simulink model "main_model"  (R2023a)
settings: Solver=ode15s  StartTime=0.0  StopTime=4  FixedStep=0.0001  RelTol=1e-3  AbsTol=1e-3  EnableMultiTasking=on
model workspace (MAT data in the model file):
  C_Gimbal = 0.5
  C_IAP = 0.01
  K_Gimbal = 0
  K_IAP = 200
  a = 1
  b = 1
  muscle_color = [0 0 1]
  muscle_radius = 1
undefined symbols (not defined in the file): X, Y, Z
libraries: nesl_utility x346, sm_lib x329, simulink_extras x33
(part 5 of 11)

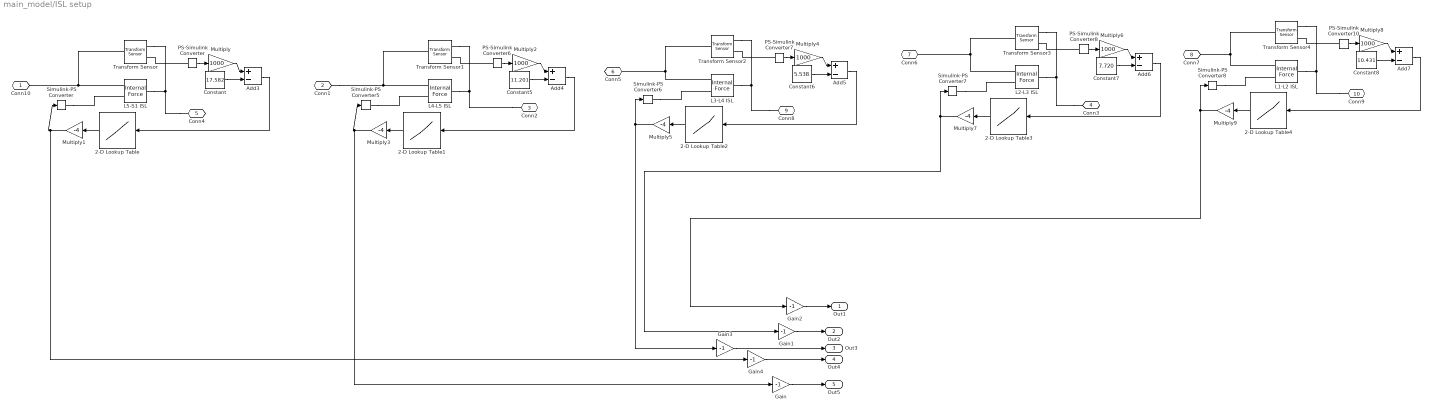
== system main_model/ISL setup ==
  2-D Lookup Table : Lookup_n-D  NumberOfTableDimensions=1  BreakpointsForDimension1=[0;0.1802;1.802;3.604;10.812]  BreakpointsForDimension2=[1:3]  Table=[0;0;4.82625;10.53;48.2625]  InternalRulePriority=Speed  RndMeth=Simplest
  2-D Lookup Table1 : Lookup_n-D  NumberOfTableDimensions=1  BreakpointsForDimension1=[0;0.1802;1.802;3.604;10.812]  BreakpointsForDimension2=[1:3]  Table=[0;0;4.82625;10.53;48.2625]  InternalRulePriority=Speed  RndMeth=Simplest
  2-D Lookup Table2 : Lookup_n-D  NumberOfTableDimensions=1  BreakpointsForDimension1=[0;0.054;0.54;1.08;3.24]  BreakpointsForDimension2=[1:3]  Table=[0;0;4.82625;10.53;48.2625]  InternalRulePriority=Speed  RndMeth=Simplest
  2-D Lookup Table3 : Lookup_n-D  NumberOfTableDimensions=1  BreakpointsForDimension1=[0;0.071;0.71;1.42;4.26]  BreakpointsForDimension2=[1:3]  Table=[0;0;4.82625;10.53;48.2625]  InternalRulePriority=Speed  RndMeth=Simplest
  2-D Lookup Table4 : Lookup_n-D  NumberOfTableDimensions=1  BreakpointsForDimension1=[0;0.105;1.05;2.1;6.3]  BreakpointsForDimension2=[1:3]  Table=[0;0;4.82625;10.53;48.2625]  InternalRulePriority=Speed  RndMeth=Simplest
  Add{3..7} (5 alike) : Sum  Inputs=+-
  Constant : Constant  Value=17.582
  Constant5 : Constant  Value=11.201
  Constant6 : Constant  Value=5.538
  Constant7 : Constant  Value=7.720
  Constant8 : Constant  Value=10.431
  Gain{,1..4} (5 alike) : Gain  Gain=-1
  L1-L2 ISL : sm_lib/Forces and Torques/Internal Force
  L2-L3 ISL : sm_lib/Forces and Torques/Internal Force
  L3-L4 ISL : sm_lib/Forces and Torques/Internal Force
  L4-L5 ISL : sm_lib/Forces and Torques/Internal Force
  L5-S1 ISL : sm_lib/Forces and Torques/Internal Force
  Multiply{,2,4,6,8} (5 alike) : Gain  Gain=1000
  Multiply{1,3,5,7,9} (5 alike) : Gain  Gain=-4
  PS-Simulink Converter{,6..8,10} (5 alike) : nesl_utility/PS-Simulink Converter  PhysicalDomain=network_engine_domain  SubClassName=ps_output  LeftPortType=input  RightPortType=output  PseudoPeriodic=off  Frequencies=[]  VectorFormat=inherit  Unit=inherit  AffineConversion=off
  Simulink-PS Converter{,5..8} (5 alike) : nesl_utility/Simulink-PS Converter  PhysicalDomain=network_engine_domain  SubClassName=ps_input  LeftPortType=input  RightPortType=output  PseudoPeriodic=off  Frequencies=[]  NoiseDistribution=none  NoiseParameters=[]  Unit=1  AffineConversion=off  FilteringAndDerivatives=provide  SimscapeFilterOrder=1  InputFilterTimeConstant=0.001  UdotUserProvided=0
  Transform Sensor{,1..4} (5 alike) : sm_lib/Frames and Transforms/Transform Sensor  MeasurementFrame=World  RotationSequence=XYX  SenseAngle=off  SenseAxis=off  SenseQ=off  SenseR=off  SenseRotationSequence=off  SenseOmegaX=off  SenseOmegaY=off  SenseOmegaZ=off  SenseQDot=off  SenseRDot=off  SenseRotationSequenceDot=off  SenseAlphaX=off  SenseAlphaY=off  SenseAlphaZ=off  SenseQDDot=off  SenseRDDot=off  SenseX=off  SenseY=off  SenseZ=off  SenseRad=off  SenseAzim=off  SenseDist=on  SenseInc=off  SenseXDot=off  SenseYDot=off  SenseZDot=off  SenseRadDot=off  SenseAzimDot=off  SenseDistDot=off  SenseIncDot=off  SenseXDDot=off  SenseYDDot=off  SenseZDDot=off  SenseRadDDot=off  SenseAzimDDot=off  SenseDistDDot=off  SenseIncDDot=off
  Conn10 : PMIOPort  Side=Left
  Conn1 : PMIOPort  Port=2  Side=Left
  Conn2 : PMIOPort  Port=3  Side=Left
  Conn3 : PMIOPort  Port=4  Side=Left
  Conn4 : PMIOPort  Port=5  Side=Left
  Conn5 : PMIOPort  Port=6  Side=Left
  Conn6 : PMIOPort  Port=7  Side=Left
  Conn7 : PMIOPort  Port=8  Side=Left
  Conn8 : PMIOPort  Port=9  Side=Left
  Conn9 : PMIOPort  Port=10  Side=Left
  Out1 : Outport
  Out2 : Outport  Port=2
  Out3 : Outport  Port=3
  Out4 : Outport  Port=4
  Out5 : Outport  Port=5
  wires:
  Gain/1 -> Out5/1
  Gain4/1 -> Out4/1
  Gain3/1 -> Out3/1
  Gain1/1 -> Out2/1
  Gain2/1 -> Out1/1
  Multiply5/1 -> Simulink-PS Converter6/1, Gain3/1
  2-D Lookup Table4/1 -> Multiply9/1
  PS-Simulink Converter/1 -> Multiply/1
  2-D Lookup Table3/1 -> Multiply7/1
  Add6/1 -> 2-D Lookup Table3/1
  Multiply/1 -> Add3/1
  2-D Lookup Table/1 -> Multiply1/1
  Constant7/1 -> Add6/2
  Multiply1/1 -> Simulink-PS Converter/1, Gain4/1
  Multiply8/1 -> Add7/1
  PS-Simulink Converter6/1 -> Multiply2/1
  2-D Lookup Table2/1 -> Multiply5/1
  Constant/1 -> Add3/2
  2-D Lookup Table1/1 -> Multiply3/1
  Constant6/1 -> Add5/2
  Multiply3/1 -> Simulink-PS Converter5/1, Gain/1
  Add4/1 -> 2-D Lookup Table1/1
  Multiply9/1 -> Simulink-PS Converter8/1, Gain2/1
  Constant5/1 -> Add4/2
  Multiply7/1 -> Simulink-PS Converter7/1, Gain1/1
  Multiply4/1 -> Add5/1
  Add3/1 -> 2-D Lookup Table/1
  Multiply2/1 -> Add4/1
  Add7/1 -> 2-D Lookup Table4/1
  PS-Simulink Converter7/1 -> Multiply4/1
  Constant8/1 -> Add7/2
  Add5/1 -> 2-D Lookup Table2/1
  PS-Simulink Converter10/1 -> Multiply8/1
  Multiply6/1 -> Add6/1
  PS-Simulink Converter8/1 -> Multiply6/1
  connections:
  Simulink-PS Converter5/RConn1 -- L4-L5 ISL/LConn2
  PS-Simulink Converter10/LConn1 -- Transform Sensor4/RConn2
  PS-Simulink Converter6/LConn1 -- Transform Sensor1/RConn2
  Simulink-PS Converter/RConn1 -- L5-S1 ISL/LConn2
  PS-Simulink Converter7/LConn1 -- Transform Sensor2/RConn2
  PS-Simulink Converter/LConn1 -- Transform Sensor/RConn2
  Simulink-PS Converter6/RConn1 -- L3-L4 ISL/LConn2
  PS-Simulink Converter8/LConn1 -- Transform Sensor3/RConn2
  Simulink-PS Converter8/RConn1 -- L1-L2 ISL/LConn2
  Conn5/RConn1 -- Transform Sensor2/LConn1 -- L3-L4 ISL/LConn1
  Conn4/RConn1 -- Transform Sensor/RConn1 -- L5-S1 ISL/RConn1
  Conn6/RConn1 -- Transform Sensor3/LConn1 -- L2-L3 ISL/LConn1
  Conn9/RConn1 -- Transform Sensor4/RConn1 -- L1-L2 ISL/RConn1
  Simulink-PS Converter7/RConn1 -- L2-L3 ISL/LConn2
  Conn3/RConn1 -- Transform Sensor3/RConn1 -- L2-L3 ISL/RConn1
  Conn7/RConn1 -- Transform Sensor4/LConn1 -- L1-L2 ISL/LConn1
  Conn8/RConn1 -- Transform Sensor2/RConn1 -- L3-L4 ISL/RConn1
  Conn1/RConn1 -- Transform Sensor1/LConn1 -- L4-L5 ISL/LConn1
  Conn2/RConn1 -- Transform Sensor1/RConn1 -- L4-L5 ISL/RConn1
  Conn10/RConn1 -- Transform Sensor/LConn1 -- L5-S1 ISL/LConn1

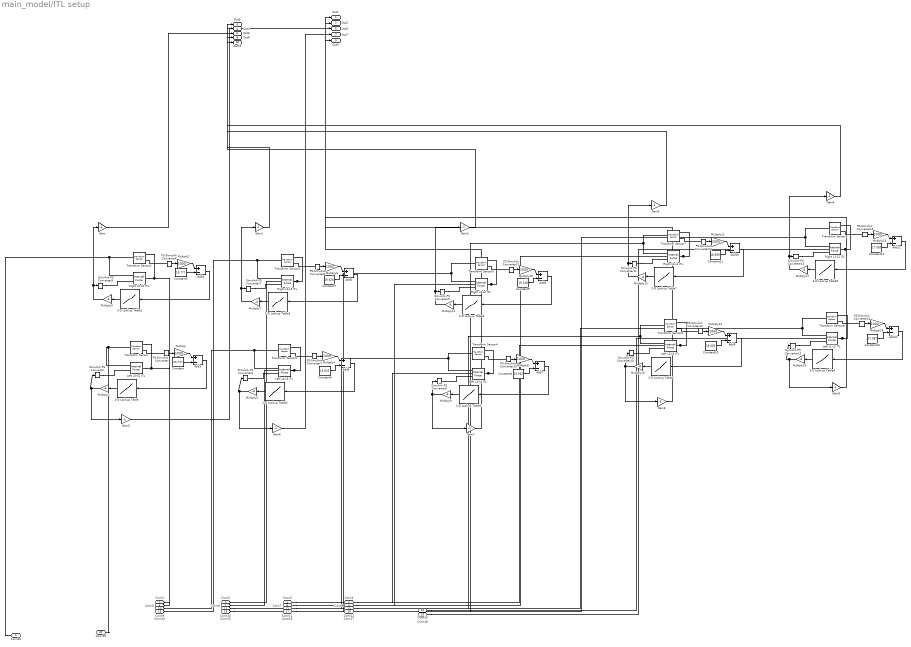
== system main_model/ITL setup ==
  2-D Lookup Table : Lookup_n-D  NumberOfTableDimensions=1  BreakpointsForDimension1=[0;0.178;2.67;3.916;5.34]  BreakpointsForDimension2=[1:3]  Table=[0;0;3;7.5;30]  InternalRulePriority=Speed  RndMeth=Simplest
  2-D Lookup Table1 : Lookup_n-D  NumberOfTableDimensions=1  BreakpointsForDimension1=[0;0.178;2.67;3.916;5.34]  BreakpointsForDimension2=[1:3]  Table=[0;0;3;7.5;30]  InternalRulePriority=Speed  RndMeth=Simplest
  2-D Lookup Table2 : Lookup_n-D  NumberOfTableDimensions=1  BreakpointsForDimension1=[0;0.213;3.195;4.686;6.39]  BreakpointsForDimension2=[1:3]  Table=[0;0;3;7.5;30]  InternalRulePriority=Speed  RndMeth=Simplest
  2-D Lookup Table3 : Lookup_n-D  NumberOfTableDimensions=1  BreakpointsForDimension1=[0;0.213;3.195;4.686;6.39]  BreakpointsForDimension2=[1:3]  Table=[0;0;3;7.5;30]  InternalRulePriority=Speed  RndMeth=Simplest
  2-D Lookup Table4 : Lookup_n-D  NumberOfTableDimensions=1  BreakpointsForDimension1=[0;0.1985;2.9775;4.367;5.955]  BreakpointsForDimension2=[1:3]  Table=[0;0;3;7.5;30]  InternalRulePriority=Speed  RndMeth=Simplest
  2-D Lookup Table5 : Lookup_n-D  NumberOfTableDimensions=1  BreakpointsForDimension1=[0;0.1985;2.9775;4.367;5.955]  BreakpointsForDimension2=[1:3]  Table=[0;0;3;7.5;30]  InternalRulePriority=Speed  RndMeth=Simplest
  2-D Lookup Table6 : Lookup_n-D  NumberOfTableDimensions=1  BreakpointsForDimension1=[0;0.2084;3.126;4.5848;6.252]  BreakpointsForDimension2=[1:3]  Table=[0;0;3;7.5;30]  InternalRulePriority=Speed  RndMeth=Simplest
  2-D Lookup Table7 : Lookup_n-D  NumberOfTableDimensions=1  BreakpointsForDimension1=[0;0.2084;3.126;4.5848;6.252]  BreakpointsForDimension2=[1:3]  Table=[0;0;3;7.5;30]  InternalRulePriority=Speed  RndMeth=Simplest
  2-D Lookup Table8 : Lookup_n-D  NumberOfTableDimensions=1  BreakpointsForDimension1=[0;0.1966;2.949;4.3252;5.898]  BreakpointsForDimension2=[1:3]  Table=[0;0;3;7.5;30]  InternalRulePriority=Speed  RndMeth=Simplest
  2-D Lookup Table9 : Lookup_n-D  NumberOfTableDimensions=1  BreakpointsForDimension1=[0;0.1966;2.949;4.3252;5.898]  BreakpointsForDimension2=[1:3]  Table=[0;0;3;7.5;30]  InternalRulePriority=Speed  RndMeth=Simplest
  Add{3..12} (10 alike) : Sum  Inputs=+-
  Constant : Constant  Value=15.777
  Constant10 : Constant  Value=18.659
  Constant11 : Constant  Value=18.659
  Constant12 : Constant  Value=17.087
  Constant13 : Constant  Value=17.087
  Constant5 : Constant  Value=15.777
  Constant6 : Constant  Value=19.625
  Constant7 : Constant  Value=19.625
  Constant8 : Constant  Value=19.562
  Constant9 : Constant  Value=19.248
  Gain{,1..9} (10 alike) : Gain  Gain=-1
  Left L1-L2 ITL : sm_lib/Forces and Torques/Internal Force
  Left L2-L3 ITL : sm_lib/Forces and Torques/Internal Force
  Left L3-L4 ITL : sm_lib/Forces and Torques/Internal Force
  Left L4-L5 ITL : sm_lib/Forces and Torques/Internal Force
  Left L5-S1 ITL : sm_lib/Forces and Torques/Internal Force
  Multiply{,2,4,6,8,10,12,14,16,18} (10 alike) : Gain  Gain=1000
  Multiply{1,3,5,7,9,11,13,15,17,19} (10 alike) : Gain  Gain=-4
  PS-Simulink Converter{,6..8,10..15} (10 alike) : nesl_utility/PS-Simulink Converter  PhysicalDomain=network_engine_domain  SubClassName=ps_output  LeftPortType=input  RightPortType=output  PseudoPeriodic=off  Frequencies=[]  VectorFormat=inherit  Unit=inherit  AffineConversion=off
  Right L1-L2 ITL : sm_lib/Forces and Torques/Internal Force
  Right L2-L3 ITL : sm_lib/Forces and Torques/Internal Force
  Right L3-L4 ITL : sm_lib/Forces and Torques/Internal Force
  Right L4-L5 ITL : sm_lib/Forces and Torques/Internal Force
  Right L5-S1 ITL : sm_lib/Forces and Torques/Internal Force
  Simulink-PS Converter{,5..13} (10 alike) : nesl_utility/Simulink-PS Converter  PhysicalDomain=network_engine_domain  SubClassName=ps_input  LeftPortType=input  RightPortType=output  PseudoPeriodic=off  Frequencies=[]  NoiseDistribution=none  NoiseParameters=[]  Unit=1  AffineConversion=off  FilteringAndDerivatives=provide  SimscapeFilterOrder=1  InputFilterTimeConstant=0.001  UdotUserProvided=0
  Transform Sensor{,1..9} (10 alike) : sm_lib/Frames and Transforms/Transform Sensor  MeasurementFrame=World  RotationSequence=XYX  SenseAngle=off  SenseAxis=off  SenseQ=off  SenseR=off  SenseRotationSequence=off  SenseOmegaX=off  SenseOmegaY=off  SenseOmegaZ=off  SenseQDot=off  SenseRDot=off  SenseRotationSequenceDot=off  SenseAlphaX=off  SenseAlphaY=off  SenseAlphaZ=off  SenseQDDot=off  SenseRDDot=off  SenseX=off  SenseY=off  SenseZ=off  SenseRad=off  SenseAzim=off  SenseDist=on  SenseInc=off  SenseXDot=off  SenseYDot=off  SenseZDot=off  SenseRadDot=off  SenseAzimDot=off  SenseDistDot=off  SenseIncDot=off  SenseXDDot=off  SenseYDDot=off  SenseZDDot=off  SenseRadDDot=off  SenseAzimDDot=off  SenseDistDDot=off  SenseIncDDot=off
  Conn20 : PMIOPort  Side=Left
  Conn1 : PMIOPort  Port=2  Side=Left
  Conn2 : PMIOPort  Port=3  Side=Left
  Conn3 : PMIOPort  Port=4  Side=Left
  Conn4 : PMIOPort  Port=5  Side=Left
  Conn5 : PMIOPort  Port=6  Side=Left
  Conn6 : PMIOPort  Port=7  Side=Left
  Conn7 : PMIOPort  Port=8  Side=Left
  Conn8 : PMIOPort  Port=9  Side=Left
  Conn9 : PMIOPort  Port=10  Side=Left
  Conn10 : PMIOPort  Port=11  Side=Left
  Conn11 : PMIOPort  Port=12  Side=Left
  Conn12 : PMIOPort  Port=13  Side=Left
  Conn13 : PMIOPort  Port=14  Side=Left
  Conn14 : PMIOPort  Port=15  Side=Left
  Conn15 : PMIOPort  Port=16  Side=Left
  Conn16 : PMIOPort  Port=17  Side=Left
  Conn17 : PMIOPort  Port=18  Side=Left
  Conn18 : PMIOPort  Port=19  Side=Left
  Conn19 : PMIOPort  Port=20  Side=Left
  Out1 : Outport
  Out2 : Outport  Port=2
  Out3 : Outport  Port=3
  Out4 : Outport  Port=4
  Out5 : Outport  Port=5
  Out6 : Outport  Port=6
  Out7 : Outport  Port=7
  Out8 : Outport  Port=8
  Out9 : Outport  Port=9
  Out10 : Outport  Port=10
  wires:
  Gain5/1 -> Out5/1
  Gain6/1 -> Out7/1
  Gain8/1 -> Out2/1
  Gain9/1 -> Out1/1
  Gain/1 -> Out6/1
  Add12/1 -> 2-D Lookup Table8/1
  Gain3/1 -> Out4/1
  PS-Simulink Converter10/1 -> Multiply8/1
  Gain7/1 -> Out9/1
  2-D Lookup Table9/1 -> Multiply17/1
  PS-Simulink Converter7/1 -> Multiply4/1
  Constant8/1 -> Add7/2
  Gain4/1 -> Out3/1
  Constant11/1 -> Add10/2
  2-D Lookup Table3/1 -> Multiply7/1
  Multiply7/1 -> Simulink-PS Converter7/1, Gain1/1
  2-D Lookup Table8/1 -> Multiply19/1
  Multiply6/1 -> Add6/1
  Add8/1 -> 2-D Lookup Table5/1
  2-D Lookup Table/1 -> Multiply1/1
  Multiply4/1 -> Add5/1
  Add6/1 -> 2-D Lookup Table3/1
  Gain1/1 -> Out8/1
  Multiply16/1 -> Add11/1
  Multiply15/1 -> Simulink-PS Converter10/1, Gain8/1
  PS-Simulink Converter6/1 -> Multiply2/1
  Constant12/1 -> Add12/2
  Add3/1 -> 2-D Lookup Table/1
  Constant7/1 -> Add6/2
  2-D Lookup Table1/1 -> Multiply3/1
  2-D Lookup Table2/1 -> Multiply5/1
  Multiply8/1 -> Add7/1
  Constant9/1 -> Add8/2
  Add4/1 -> 2-D Lookup Table1/1
  Constant6/1 -> Add5/2
  Add11/1 -> 2-D Lookup Table9/1
  PS-Simulink Converter15/1 -> Multiply16/1
  PS-Simulink Converter13/1 -> Multiply12/1
  2-D Lookup Table4/1 -> Multiply9/1
  Constant5/1 -> Add4/2
  2-D Lookup Table7/1 -> Multiply13/1
  Multiply14/1 -> Add9/1
  Multiply/1 -> Add3/1
  PS-Simulink Converter8/1 -> Multiply6/1
  Add10/1 -> 2-D Lookup Table7/1
  Constant/1 -> Add3/2
  Gain2/1 -> Out10/1
  Multiply13/1 -> Simulink-PS Converter11/1, Gain3/1
  Multiply12/1 -> Add10/1
  PS-Simulink Converter14/1 -> Multiply18/1
  Multiply10/1 -> Add8/1
  Multiply17/1 -> Simulink-PS Converter13/1, Gain4/1
  PS-Simulink Converter/1 -> Multiply/1
  2-D Lookup Table5/1 -> Multiply11/1
  Multiply2/1 -> Add4/1
  Multiply11/1 -> Simulink-PS Converter9/1, Gain2/1
  Multiply19/1 -> Simulink-PS Converter12/1, Gain9/1
  Add9/1 -> 2-D Lookup Table6/1
  Multiply18/1 -> Add12/1
  Constant10/1 -> Add9/2
  PS-Simulink Converter11/1 -> Multiply10/1
  Multiply1/1 -> Simulink-PS Converter/1, Gain5/1
  Multiply3/1 -> Simulink-PS Converter5/1, Gain/1
  Multiply9/1 -> Gain7/1, Simulink-PS Converter8/1
  Add5/1 -> 2-D Lookup Table2/1
  Add7/1 -> 2-D Lookup Table4/1
  Constant13/1 -> Add11/2
  PS-Simulink Converter12/1 -> Multiply14/1
  Multiply5/1 -> Simulink-PS Converter6/1, Gain6/1
  2-D Lookup Table6/1 -> Multiply15/1
  connections:
  PS-Simulink Converter8/LConn1 -- Transform Sensor3/RConn2
  PS-Simulink Converter11/LConn1 -- Transform Sensor5/RConn2
  Simulink-PS Converter12/RConn1 -- Left L1-L2 ITL/LConn2
  Conn14/RConn1 -- Right L4-L5 ITL/LConn1 -- Transform Sensor3/LConn1
  Simulink-PS Converter7/RConn1 -- Right L4-L5 ITL/LConn2
  Conn1/RConn1 -- Transform Sensor/RConn1 -- Left L5-S1 ITL/RConn1
  Conn10/RConn1 -- Left L3-L4 ITL/LConn1 -- Transform Sensor4/LConn1
  Simulink-PS Converter11/RConn1 -- Right L2-L3 ITL/LConn2
  Simulink-PS Converter10/RConn1 -- Left L2-L3 ITL/LConn2
  Conn12/RConn1 -- Left L1-L2 ITL/LConn1 -- Transform Sensor8/LConn1
  Simulink-PS Converter9/RConn1 -- Right L3-L4 ITL/LConn2
  PS-Simulink Converter7/LConn1 -- Transform Sensor2/RConn2
  PS-Simulink Converter6/LConn1 -- Transform Sensor1/RConn2
  Conn8/RConn1 -- Transform Sensor7/RConn1 -- Right L2-L3 ITL/RConn1
  PS-Simulink Converter14/LConn1 -- Transform Sensor8/RConn2
  Simulink-PS Converter13/RConn1 -- Right L1-L2 ITL/LConn2
  Conn3/RConn1 -- Transform Sensor4/RConn1 -- Left L3-L4 ITL/RConn1
  Conn18/RConn1 -- Transform Sensor9/RConn1 -- Right L1-L2 ITL/RConn1
  PS-Simulink Converter15/LConn1 -- Transform Sensor9/RConn2
  Simulink-PS Converter6/RConn1 -- Left L4-L5 ITL/LConn2
  Conn17/RConn1 -- Right L1-L2 ITL/LConn1 -- Transform Sensor9/LConn1
  Conn15/RConn1 -- Right L3-L4 ITL/LConn1 -- Transform Sensor5/LConn1
  PS-Simulink Converter12/LConn1 -- Transform Sensor6/RConn2
  Conn7/RConn1 -- Transform Sensor5/RConn1 -- Right L3-L4 ITL/RConn1
  Simulink-PS Converter5/RConn1 -- Right L5-S1 ITL/LConn2
  Conn13/RConn1 -- Transform Sensor8/RConn1 -- Left L1-L2 ITL/RConn1
  PS-Simulink Converter/LConn1 -- Transform Sensor/RConn2
  Conn11/RConn1 -- Left L2-L3 ITL/LConn1 -- Transform Sensor6/LConn1
  Simulink-PS Converter8/RConn1 -- Left L3-L4 ITL/LConn2
  Conn5/RConn1 -- Transform Sensor1/RConn1 -- Right L5-S1 ITL/RConn1
  Conn19/RConn1 -- Transform Sensor/LConn1 -- Left L5-S1 ITL/LConn1
  Conn4/RConn1 -- Transform Sensor6/RConn1 -- Left L2-L3 ITL/RConn1
  Conn20/RConn1 -- Right L5-S1 ITL/LConn1 -- Transform Sensor1/LConn1
  Conn9/RConn1 -- Left L4-L5 ITL/LConn1 -- Transform Sensor2/LConn1
  Conn16/RConn1 -- Right L2-L3 ITL/LConn1 -- Transform Sensor7/LConn1
  Conn6/RConn1 -- Transform Sensor2/RConn1 -- Left L4-L5 ITL/RConn1
  Conn2/RConn1 -- Transform Sensor3/RConn1 -- Right L4-L5 ITL/RConn1
  Simulink-PS Converter/RConn1 -- Left L5-S1 ITL/LConn2
  PS-Simulink Converter13/LConn1 -- Transform Sensor7/RConn2
  PS-Simulink Converter10/LConn1 -- Transform Sensor4/RConn2

== system main_model/L1 ==
  AR torque feedback L4 : Subsystem
  FE torque feedback L4 : Subsystem
  File Solid : sm_lib/Body Elements/File Solid  ExtGeomFileName=C:\Users\siril\OneDrive\Desktop\TIM-Control\Matlab\Simscape models\CAD - with COM\SymmetricModel\draft7\L1.step  UnitType=FromFile  ExtGeomFileUnits=m  StepReaderType=HEX  ExportConvexHullGeometry=off  InertiaType=CalculateFromGeometry  Mass=1  MassUnits=kg  CenterOfMass=[0 0 0]  CenterOfMassUnits=m  MomentsOfInertia=[1 1 1]  MomentsOfInertiaUnits=kg*m^2  ProductsOfInertia=[0 0 0]  ProductsOfInertiaUnits=kg*m^2  BasedOnType=Density  Density=0.182  DensityUnits=g/cm^3  DoExposeReferenceFrame=on  SerializedFrames=<Frames><Frame><Id>Frame1</Id><Value><Name>To L2</Name><Origin><Source>GeometricFeature</Source><FeatureName>planar surface 2992</FeatureName></Origin><PrimaryAxis><DefinedDirection>+Z</DefinedDirection><Source>GeometricFeature</Source><SourceDirection>+Z</SourceDirection><FeatureName>planar surface 2992</FeatureName></PrimaryAxis><SecondaryAxis><DefinedDirection>+X</DefinedDirection><Source>ReferenceFrame</Source><SourceDirection>+X</SourceDirection><FeatureName></FeatureName></SecondaryAxis></Value></Frame><Frame><Id>Frame2</Id><Value><Name>To T12</Name><Origin><Source>GeometricFeature</Source><FeatureName>segment 4586</FeatureName></Origin><PrimaryAxis><DefinedDirection>+Z</DefinedDirection><Source>GeometricFeature</Source><SourceDirection>+Z</SourceDirection><FeatureName>planar surface 2965</FeatureName></PrimaryAxis><SecondaryAxis><DefinedDirection>+X</DefinedDirection><Source>ReferenceFrame</Source><SourceDirection>+X</SourceDirection><FeatureName></FeatureName></SecondaryAxis></Value></Frame><Frame><Id>Frame3</Id><Value><Name>L1 COM</Name><Origin><Source>CenterOfMassFrame</Source><FeatureName></FeatureName></Origin><PrimaryAxis><DefinedDirection>+Z</DefinedDirection><Source>ReferenceFrame</Source><SourceDirection>+Z</SourceDirection><FeatureName></FeatureName></PrimaryAxis><SecondaryAxis><DefinedDirection>+X</DefinedDirection><Source>ReferenceFrame</Source><SourceDirection>+X</SourceDirection><FeatureName></FeatureName></SecondaryAxis></Value></Frame><Frame><Id>Frame4</Id><Value><Name>L1 Abd Force</Name><Origin><Source>GeometricFeature</Source><FeatureName>point 2</FeatureName></Origin><PrimaryAxis><DefinedDirection>+Z</DefinedDirection><Source>GeometricFeature</Source><SourceDirection>+Z</SourceDirection><FeatureName>conical surface 2</FeatureName></PrimaryAxis><SecondaryAxis><DefinedDirection>+X</DefinedDirection><Source>ReferenceFrame</Source><SourceDirection>+X</SourceDirection><FeatureName></FeatureName></SecondaryAxis></Value></Frame><Frame><Id>Frame5</Id><Value><Name>To L2 ISL</Name><Origin><Source>GeometricFeature</Source><FeatureName>point 8203</FeatureName></Origin><PrimaryAxis><DefinedDirection>+Z</DefinedDirection><Source>ReferenceFrame</Source><SourceDirection>+Z</SourceDirection><FeatureName></FeatureName></PrimaryAxis><SecondaryAxis><DefinedDirection>+X</DefinedDirection><Source>ReferenceFrame</Source><SourceDirection>+X</SourceDirection><FeatureName></FeatureName></SecondaryAxis></Value></Frame><Frame><Id>Frame6</Id><Value><Name>To L2 SSL</Name><Origin><Source>GeometricFeature</Source><FeatureName>point 7953</FeatureName></Origin><PrimaryAxis><DefinedDirection>+Z</DefinedDirection><Source>ReferenceFrame</Source><SourceDirection>+Z</SourceDirection><FeatureName></FeatureName></PrimaryAxis><SecondaryAxis><DefinedDirection>+X</DefinedDirection><Source>ReferenceFrame</Source><SourceDirection>+X</SourceDirection><FeatureName></FeatureName></SecondaryAxis></Value></Frame><Frame><Id>Frame7</Id><Value><Name>To Left L2 ITL</Name><Origin><Source>GeometricFeature</Source><FeatureName>point 8094</FeatureName></Origin><PrimaryAxis><DefinedDirection>+Z</DefinedDirection><Source>ReferenceFrame</Source><SourceDirection>+Z</SourceDirection><FeatureName></FeatureName></PrimaryAxis><SecondaryAxis><DefinedDirection>+X</DefinedDirection><Source>ReferenceFrame</Source><SourceDirection>+X</SourceDirection><FeatureName></FeatureName></SecondaryAxis></Value></Frame><Frame><Id>Frame8</Id><Value><Name>To Right L2 ITL</Name><Origin><Source>GeometricFeature</Source><FeatureName>point 3432</FeatureName></Origin><PrimaryAxis><DefinedDirection>+Z</DefinedDirection><Source>ReferenceFrame</Source><SourceDirection>+Z</SourceDirection><FeatureName></FeatureName></PrimaryAxis><SecondaryAxis><DefinedDirection>+X</DefinedDirection><Source>ReferenceFrame</Source><SourceDirection>+X</SourceDirection><FeatureName></FeatureName></SecondaryAxis></Value></Frame></Frames>  GraphicType=FromGeometry  MarkerShape=Sphere  MarkerSize=10  GraphicVisPropType=SimpleVisualProperties  GraphicDiffuseColor=[0.8901961 0.85490197 0.7882353]  GraphicSpecularColor=[0.5 0.5 0.5 1.0]  GraphicAmbientColor=[0.15 0.15 0.15 1.0]  GraphicEmissiveColor=[0.0 0.0 0.0 1.0]  GraphicShininess=75  GraphicOpacity=1.0
  Gimbal Joint1 : sm_lib/Joints/Gimbal Joint  JointMode=Normal  SenseConstraintForce=off  SenseConstraintForceX=off  SenseConstraintForceY=off  SenseConstraintForceZ=off  SenseConstraintTorque=off  SenseConstraintTorqueX=off  SenseConstraintTorqueY=off  SenseConstraintTorqueZ=off  SenseTotalForce=off  SenseTotalForceX=off  SenseTotalForceY=off  SenseTotalForceZ=off  SenseTotalTorque=off  SenseTotalTorqueX=off  SenseTotalTorqueY=off  SenseTotalTorqueZ=off  CompositeWrenchDir=FollowerOnBase  CompositeWrenchFrame=BaseFrame  RxEquilibriumPosition=0  RxEquilibriumPositionUnits=deg  RxSpringStiffness=K_Gimbal  RxSpringStiffnessUnits=N*m/deg  RxDampingCoefficient=C_Gimbal  RxDampingCoefficientUnits=N*m/(deg/s)  RxTorqueActuationMode=InputTorque  RxMotionActuationMode=ComputedMotion  RxSensePosition=on  RxSenseVelocity=off  RxSenseAcceleration=off  RxSenseTorqueForce=on  RxSenseLowerLimitTorqueForce=off  RxSenseUpperLimitTorqueForce=off  RxLowerLimitSpecify=on  RxLowerLimitBound=-30  RxLowerLimitBoundUnits=deg  RxLowerLimitStiffness=10000  RxLowerLimitStiffnessUnits=N*m/deg  RxLowerLimitDamping=100  RxLowerLimitDampingUnits=N*m/(deg/s)  RxLowerLimitTransitionRegionWidth=0.1  RxLowerLimitTransitionRegionWidthUnits=deg  RxUpperLimitSpecify=on  RxUpperLimitBound=30  RxUpperLimitBoundUnits=deg  RxUpperLimitStiffness=10000  RxUpperLimitStiffnessUnits=N*m/deg  RxUpperLimitDamping=100  RxUpperLimitDampingUnits=N*m/(deg/s)  RxUpperLimitTransitionRegionWidth=0.1  RxUpperLimitTransitionRegionWidthUnits=deg  RxPositionTargetSpecify=off  RxPositionTargetPriority=High  RxPositionTargetValue=0  RxPositionTargetValueUnits=deg  RxVelocityTargetSpecify=off  RxVelocityTargetPriority=High  RxVelocityTargetValue=0  RxVelocityTargetValueUnits=deg/s  RyEquilibriumPosition=0  RyEquilibriumPositionUnits=deg  RySpringStiffness=K_Gimbal  RySpringStiffnessUnits=N*m/deg  RyDampingCoefficient=C_Gimbal  RyDampingCoefficientUnits=N*m/(deg/s)  RyTorqueActuationMode=InputTorque  RyMotionActuationMode=ComputedMotion  RySensePosition=on  RySenseVelocity=off  RySenseAcceleration=off  RySenseTorqueForce=on  RySenseLowerLimitTorqueForce=off  RySenseUpperLimitTorqueForce=off  RyLowerLimitSpecify=on  RyLowerLimitBound=-30  RyLowerLimitBoundUnits=deg  RyLowerLimitStiffness=10000  RyLowerLimitStiffnessUnits=N*m/deg  RyLowerLimitDamping=100  RyLowerLimitDampingUnits=N*m/(deg/s)  RyLowerLimitTransitionRegionWidth=0.1  RyLowerLimitTransitionRegionWidthUnits=deg  RyUpperLimitSpecify=on  RyUpperLimitBound=30  RyUpperLimitBoundUnits=deg  RyUpperLimitStiffness=10000  RyUpperLimitStiffnessUnits=N*m/deg  RyUpperLimitDamping=100  RyUpperLimitDampingUnits=N*m/(deg/s)  RyUpperLimitTransitionRegionWidth=0.1  RyUpperLimitTransitionRegionWidthUnits=deg  RyPositionTargetSpecify=off  RyPositionTargetPriority=High  RyPositionTargetValue=0  RyPositionTargetValueUnits=deg  RyVelocityTargetSpecify=off  RyVelocityTargetPriority=High  RyVelocityTargetValue=0  RyVelocityTargetValueUnits=deg/s  RzEquilibriumPosition=0  RzEquilibriumPositionUnits=deg  RzSpringStiffness=K_Gimbal  RzSpringStiffnessUnits=N*m/deg  RzDampingCoefficient=C_Gimbal  RzDampingCoefficientUnits=N*m/(deg/s)  RzTorqueActuationMode=InputTorque  RzMotionActuationMode=ComputedMotion  RzSensePosition=on  RzSenseVelocity=off  RzSenseAcceleration=off  RzSenseTorqueForce=on  RzSenseLowerLimitTorqueForce=off  RzSenseUpperLimitTorqueForce=off  RzLowerLimitSpecify=on  RzLowerLimitBound=-30  RzLowerLimitBoundUnits=deg  RzLowerLimitStiffness=10000  RzLowerLimitStiffnessUnits=N*m/deg  RzLowerLimitDamping=100  RzLowerLimitDampingUnits=N*m/(deg/s)  RzLowerLimitTransitionRegionWidth=0.1  RzLowerLimitTransitionRegionWidthUnits=deg  RzUpperLimitSpecify=on  RzUpperLimitBound=30  RzUpperLimitBoundUnits=deg  RzUpperLimitStiffness=10000  RzUpperLimitStiffnessUnits=N*m/deg  RzUpperLimitDamping=100  RzUpperLimitDampingUnits=N*m/(deg/s)  RzUpperLimitTransitionRegionWidth=0.1  RzUpperLimitTransitionRegionWidthUnits=deg  RzPositionTargetSpecify=off  RzPositionTargetPriority=High  RzPositionTargetValue=0  RzPositionTargetValueUnits=deg  RzVelocityTargetSpecify=off  RzVelocityTargetPriority=High  RzVelocityTargetValue=0  RzVelocityTargetValueUnits=deg/s
  LB torque feedback L4 : Subsystem
  to L2 : PMIOPort  Side=Left
  to T12 : PMIOPort  Port=2  Side=Right
  FE rot : PMIOPort  Port=3  Side=Right
  FE torque : PMIOPort  Port=4  Side=Right
  LB rot : PMIOPort  Port=5  Side=Right
  LB torque : PMIOPort  Port=6  Side=Right
  AR rot : PMIOPort  Port=7  Side=Right
  AR torque : PMIOPort  Port=8  Side=Right
  L1 COM : PMIOPort  Port=9  Side=Right
  L1 Abd Force : PMIOPort  Port=10  Side=Right
  To L2 ISL : PMIOPort  Port=11  Side=Right
  To L2 SSL : PMIOPort  Port=12  Side=Right
  To Left L2 ITL : PMIOPort  Port=13  Side=Right
  To Right L2 ITL : PMIOPort  Port=14  Side=Right
  connections:
  To Right L2 ITL/RConn1 -- File Solid/LConn5
  To Left L2 ITL/RConn1 -- File Solid/RConn4
  To L2 SSL/RConn1 -- File Solid/LConn4
  To L2 ISL/RConn1 -- File Solid/RConn3
  L1 Abd Force/RConn1 -- File Solid/LConn3
  L1 COM/RConn1 -- File Solid/RConn2
  AR torque/RConn1 -- Gimbal Joint1/RConn7
  LB torque/RConn1 -- Gimbal Joint1/RConn5
  FE torque/RConn1 -- Gimbal Joint1/RConn3
  Gimbal Joint1/LConn4 -- AR torque feedback L4/RConn1
  Gimbal Joint1/LConn3 -- LB torque feedback L4/RConn1
  Gimbal Joint1/LConn2 -- FE torque feedback L4/RConn1
  AR torque feedback L4/LConn1 -- AR rot/RConn1 -- Gimbal Joint1/RConn6
  LB torque feedback L4/LConn1 -- LB rot/RConn1 -- Gimbal Joint1/RConn4
  FE rot/RConn1 -- FE torque feedback L4/LConn1 -- Gimbal Joint1/RConn2
  Gimbal Joint1/RConn1 -- File Solid/LConn1
  to T12/RConn1 -- File Solid/LConn2
  Gimbal Joint1/LConn1 -- to L2/RConn1

== system main_model/L1 moment setup ==
  input0 : Inport
  input1 : Inport  Port=2
  input2 : Inport  Port=3
  input3 : Inport  Port=4
  Flexion force at T1 : sm_lib/Forces and Torques/External Force and Torque  ForceResolutionFrame=AttachedFrame  EnableForceX=off  EnableForceY=on  EnableForceZ=off  EnableForce=off  TorqueResolutionFrame=AttachedFrame  EnableTorqueX=off  EnableTorqueY=off  EnableTorqueZ=off  EnableTorque=off
  Pure AR Moment at L1 COM : sm_lib/Forces and Torques/External Force and Torque  ForceResolutionFrame=World  EnableForceX=off  EnableForceY=off  EnableForceZ=off  EnableForce=off  TorqueResolutionFrame=World  EnableTorqueX=off  EnableTorqueY=off  EnableTorqueZ=on  EnableTorque=off
  Pure FE Moment at L1 COM : sm_lib/Forces and Torques/External Force and Torque  ForceResolutionFrame=World  EnableForceX=off  EnableForceY=off  EnableForceZ=off  EnableForce=off  TorqueResolutionFrame=World  EnableTorqueX=on  EnableTorqueY=off  EnableTorqueZ=off  EnableTorque=off
  Pure LB Moment at L1 COM : sm_lib/Forces and Torques/External Force and Torque  ForceResolutionFrame=World  EnableForceX=off  EnableForceY=off  EnableForceZ=off  EnableForce=off  TorqueResolutionFrame=World  EnableTorqueX=off  EnableTorqueY=on  EnableTorqueZ=off  EnableTorque=off
  Simulink-PS Converter{1..4} (4 alike) : nesl_utility/Simulink-PS Converter  PhysicalDomain=network_engine_domain  SubClassName=ps_input  LeftPortType=input  RightPortType=output  PseudoPeriodic=off  Frequencies=[]  NoiseDistribution=none  NoiseParameters=[]  Unit=1  AffineConversion=off  FilteringAndDerivatives=provide  SimscapeFilterOrder=1  InputFilterTimeConstant=0.001  UdotUserProvided=0
  Conn1 : PMIOPort  Side=Left
  Conn2 : PMIOPort  Port=2  Side=Right
  Out1 : Outport
  Out2 : Outport  Port=2
  Out3 : Outport  Port=3
  wires:
  input2/1 -> Simulink-PS Converter2/1, Out1/1
  input3/1 -> Simulink-PS Converter1/1
  input1/1 -> Simulink-PS Converter3/1, Out2/1
  input0/1 -> Simulink-PS Converter4/1, Out3/1
  connections:
  Simulink-PS Converter1/RConn1 -- Flexion force at T1/LConn1
  Simulink-PS Converter4/RConn1 -- Pure AR Moment at L1 COM/LConn1
  Simulink-PS Converter2/RConn1 -- Pure FE Moment at L1 COM/LConn1
  Flexion force at T1/RConn1 -- Conn2/RConn1
  Simulink-PS Converter3/RConn1 -- Pure LB Moment at L1 COM/LConn1
  Conn1/RConn1 -- Pure FE Moment at L1 COM/RConn1 -- Pure AR Moment at L1 COM/RConn1 -- Pure LB Moment at L1 COM/RConn1

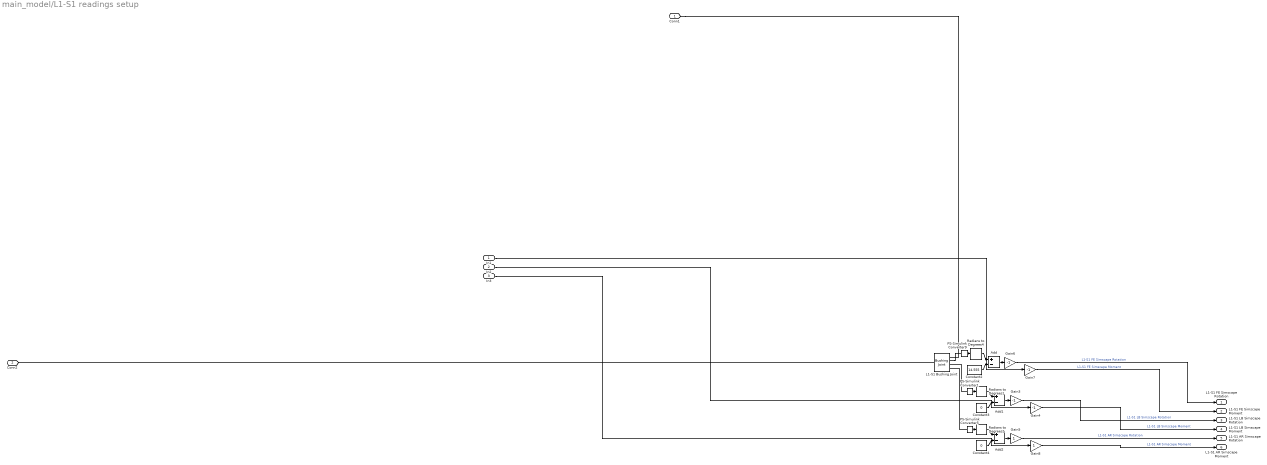
== system main_model/L1-S1 readings setup ==
  In1 : Inport
  In2 : Inport  Port=2
  In3 : Inport  Port=3
  Add : Sum  Inputs=+-
  Add1 : Sum  Inputs=+-
  Add2 : Sum  Inputs=+-
  Constant2 : Constant  Value=14.555
  Constant3 : Constant  Value=0
  Constant4 : Constant  Value=0
  Gain{3..4,6..7} (4 alike) : Gain  Gain=-1
  Gain5 : Gain
  Gain8 : Gain
  L1-S1 Bushing Joint : sm_lib/Joints/Bushing Joint  JointMode=Normal  SenseConstraintForce=off  SenseConstraintForceX=off  SenseConstraintForceY=off  SenseConstraintForceZ=off  SenseConstraintTorque=off  SenseConstraintTorqueX=off  SenseConstraintTorqueY=off  SenseConstraintTorqueZ=off  SenseTotalForce=off  SenseTotalForceX=off  SenseTotalForceY=off  SenseTotalForceZ=off  SenseTotalTorque=off  SenseTotalTorqueX=off  SenseTotalTorqueY=off  SenseTotalTorqueZ=off  CompositeWrenchDir=FollowerOnBase  CompositeWrenchFrame=FollowerFrame  PxEquilibriumPosition=0  PxEquilibriumPositionUnits=m  PxSpringStiffness=0  PxSpringStiffnessUnits=N/m  PxDampingCoefficient=0  PxDampingCoefficientUnits=N/(m/s)  PxTorqueActuationMode=NoTorque  PxMotionActuationMode=ComputedMotion  PxSensePosition=off  PxSenseVelocity=off  PxSenseAcceleration=off  PxSenseTorqueForce=off  PxSenseLowerLimitTorqueForce=off  PxSenseUpperLimitTorqueForce=off  PxLowerLimitSpecify=off  PxLowerLimitBound=-1  PxLowerLimitBoundUnits=m  PxLowerLimitStiffness=1e6  PxLowerLimitStiffnessUnits=N/m  PxLowerLimitDamping=1e3  PxLowerLimitDampingUnits=N/(m/s)  PxLowerLimitTransitionRegionWidth=1e-4  PxLowerLimitTransitionRegionWidthUnits=m  PxUpperLimitSpecify=off  PxUpperLimitBound=1  PxUpperLimitBoundUnits=m  PxUpperLimitStiffness=1e6  PxUpperLimitStiffnessUnits=N/m  PxUpperLimitDamping=1e3  PxUpperLimitDampingUnits=N/(m/s)  PxUpperLimitTransitionRegionWidth=1e-4  PxUpperLimitTransitionRegionWidthUnits=m  PxPositionTargetSpecify=off  PxPositionTargetPriority=High  PxPositionTargetValue=0  PxPositionTargetValueUnits=m  PxVelocityTargetSpecify=off  PxVelocityTargetPriority=High  PxVelocityTargetValue=0  PxVelocityTargetValueUnits=m/s  PyEquilibriumPosition=0  PyEquilibriumPositionUnits=m  PySpringStiffness=0  PySpringStiffnessUnits=N/m  PyDampingCoefficient=0  PyDampingCoefficientUnits=N/(m/s)  PyTorqueActuationMode=NoTorque  PyMotionActuationMode=ComputedMotion  PySensePosition=off  PySenseVelocity=off  PySenseAcceleration=off  PySenseTorqueForce=off  PySenseLowerLimitTorqueForce=off  PySenseUpperLimitTorqueForce=off  PyLowerLimitSpecify=off  PyLowerLimitBound=-1  PyLowerLimitBoundUnits=m  PyLowerLimitStiffness=1e6  PyLowerLimitStiffnessUnits=N/m  PyLowerLimitDamping=1e3  PyLowerLimitDampingUnits=N/(m/s)  PyLowerLimitTransitionRegionWidth=1e-4  PyLowerLimitTransitionRegionWidthUnits=m  PyUpperLimitSpecify=off  PyUpperLimitBound=1  PyUpperLimitBoundUnits=m  PyUpperLimitStiffness=1e6  PyUpperLimitStiffnessUnits=N/m  PyUpperLimitDamping=1e3  PyUpperLimitDampingUnits=N/(m/s)  PyUpperLimitTransitionRegionWidth=1e-4  PyUpperLimitTransitionRegionWidthUnits=m  PyPositionTargetSpecify=off  PyPositionTargetPriority=High  PyPositionTargetValue=0  PyPositionTargetValueUnits=m  PyVelocityTargetSpecify=off  PyVelocityTargetPriority=High  PyVelocityTargetValue=0  PyVelocityTargetValueUnits=m/s  PzEquilibriumPosition=0  PzEquilibriumPositionUnits=m  PzSpringStiffness=0  PzSpringStiffnessUnits=N/m  PzDampingCoefficient=0  PzDampingCoefficientUnits=N/(m/s)  PzTorqueActuationMode=NoTorque  PzMotionActuationMode=ComputedMotion  PzSensePosition=off  PzSenseVelocity=off  PzSenseAcceleration=off  PzSenseTorqueForce=off  PzSenseLowerLimitTorqueForce=off  PzSenseUpperLimitTorqueForce=off  PzLowerLimitSpecify=off  PzLowerLimitBound=-1  PzLowerLimitBoundUnits=m  PzLowerLimitStiffness=1e6  PzLowerLimitStiffnessUnits=N/m  PzLowerLimitDamping=1e3  PzLowerLimitDampingUnits=N/(m/s)  PzLowerLimitTransitionRegionWidth=1e-4  PzLowerLimitTransitionRegionWidthUnits=m  PzUpperLimitSpecify=off  PzUpperLimitBound=1  PzUpperLimitBoundUnits=m  PzUpperLimitStiffness=1e6  PzUpperLimitStiffnessUnits=N/m  PzUpperLimitDamping=1e3  PzUpperLimitDampingUnits=N/(m/s)  PzUpperLimitTransitionRegionWidth=1e-4  PzUpperLimitTransitionRegionWidthUnits=m  PzPositionTargetSpecify=off  PzPositionTargetPriority=High  PzPositionTargetValue=0  PzPositionTargetValueUnits=m  PzVelocityTargetSpecify=off  PzVelocityTargetPriority=High  PzVelocityTargetValue=0  PzVelocityTargetValueUnits=m/s  RxEquilibriumPosition=0  RxEquilibriumPositionUnits=deg  RxSpringStiffness=0  RxSpringStiffnessUnits=N*m/deg  RxDampingCoefficient=0  RxDampingCoefficientUnits=N*m/(deg/s)  RxTorqueActuationMode=NoTorque  RxMotionActuationMode=ComputedMotion  RxSensePosition=on  RxSenseVelocity=off  RxSenseAcceleration=off  RxSenseTorqueForce=off  RxSenseLowerLimitTorqueForce=off  RxSenseUpperLimitTorqueForce=off  RxLowerLimitSpecify=off  RxLowerLimitBound=-90  RxLowerLimitBoundUnits=deg  RxLowerLimitStiffness=1e4  RxLowerLimitStiffnessUnits=N*m/deg  RxLowerLimitDamping=10  RxLowerLimitDampingUnits=N*m/(deg/s)  RxLowerLimitTransitionRegionWidth=0.1  RxLowerLimitTransitionRegionWidthUnits=deg  RxUpperLimitSpecify=off  RxUpperLimitBound=90  RxUpperLimitBoundUnits=deg  RxUpperLimitStiffness=1e4  RxUpperLimitStiffnessUnits=N*m/deg  RxUpperLimitDamping=10  RxUpperLimitDampingUnits=N*m/(deg/s)  RxUpperLimitTransitionRegionWidth=0.1  RxUpperLimitTransitionRegionWidthUnits=deg  RxPositionTargetSpecify=off  RxPositionTargetPriority=High  RxPositionTargetValue=0  RxPositionTargetValueUnits=deg  RxVelocityTargetSpecify=off  RxVelocityTargetPriority=High  RxVelocityTargetValue=0  RxVelocityTargetValueUnits=deg/s  RyEquilibriumPosition=0  RyEquilibriumPositionUnits=deg  RySpringStiffness=0  RySpringStiffnessUnits=N*m/deg  RyDampingCoefficient=0  RyDampingCoefficientUnits=N*m/(deg/s)  RyTorqueActuationMode=NoTorque  RyMotionActuationMode=ComputedMotion  RySensePosition=on  RySenseVelocity=off  RySenseAcceleration=off  RySenseTorqueForce=off  RySenseLowerLimitTorqueForce=off  RySenseUpperLimitTorqueForce=off  RyLowerLimitSpecify=off  RyLowerLimitBound=-90  RyLowerLimitBoundUnits=deg  RyLowerLimitStiffness=1e4  RyLowerLimitStiffnessUnits=N*m/deg  RyLowerLimitDamping=10  RyLowerLimitDampingUnits=N*m/(deg/s)  RyLowerLimitTransitionRegionWidth=0.1  RyLowerLimitTransitionRegionWidthUnits=deg  RyUpperLimitSpecify=off  RyUpperLimitBound=90  RyUpperLimitBoundUnits=deg  RyUpperLimitStiffness=1e4  RyUpperLimitStiffnessUnits=N*m/deg  RyUpperLimitDamping=10  RyUpperLimitDampingUnits=N*m/(deg/s)  RyUpperLimitTransitionRegionWidth=0.1  RyUpperLimitTransitionRegionWidthUnits=deg  RyPositionTargetSpecify=off  RyPositionTargetPriority=High  RyPositionTargetValue=0  RyPositionTargetValueUnits=deg  RyVelocityTargetSpecify=off  RyVelocityTargetPriority=High  RyVelocityTargetValue=0  RyVelocityTargetValueUnits=deg/s  RzEquilibriumPosition=0  RzEquilibriumPositionUnits=deg  RzSpringStiffness=0  RzSpringStiffnessUnits=N*m/deg  RzDampingCoefficient=0  RzDampingCoefficientUnits=N*m/(deg/s)  RzTorqueActuationMode=NoTorque  RzMotionActuationMode=ComputedMotion  RzSensePosition=on  RzSenseVelocity=off  RzSenseAcceleration=off  RzSenseTorqueForce=off  RzSenseLowerLimitTorqueForce=off  RzSenseUpperLimitTorqueForce=off  RzLowerLimitSpecify=off  RzLowerLimitBound=-90  RzLowerLimitBoundUnits=deg  RzLowerLimitStiffness=1e4  RzLowerLimitStiffnessUnits=N*m/deg  RzLowerLimitDamping=10  RzLowerLimitDampingUnits=N*m/(deg/s)  RzLowerLimitTransitionRegionWidth=0.1  RzLowerLimitTransitionRegionWidthUnits=deg  RzUpperLimitSpecify=off  RzUpperLimitBound=90  RzUpperLimitBoundUnits=deg  RzUpperLimitStiffness=1e4  RzUpperLimitStiffnessUnits=N*m/deg  RzUpperLimitDamping=10  RzUpperLimitDampingUnits=N*m/(deg/s)  RzUpperLimitTransitionRegionWidth=0.1  RzUpperLimitTransitionRegionWidthUnits=deg  RzPositionTargetSpecify=off  RzPositionTargetPriority=High  RzPositionTargetValue=0  RzPositionTargetValueUnits=deg  RzVelocityTargetSpecify=off  RzVelocityTargetPriority=High  RzVelocityTargetValue=0  RzVelocityTargetValueUnits=deg/s
  PS-Simulink Converter1 : nesl_utility/PS-Simulink Converter  PhysicalDomain=network_engine_domain  SubClassName=ps_output  LeftPortType=input  RightPortType=output  PseudoPeriodic=off  Frequencies=[]  VectorFormat=inherit  Unit=inherit  AffineConversion=off
  PS-Simulink Converter5 : nesl_utility/PS-Simulink Converter  PhysicalDomain=network_engine_domain  SubClassName=ps_output  LeftPortType=input  RightPortType=output  PseudoPeriodic=off  Frequencies=[]  VectorFormat=inherit  Unit=inherit  AffineConversion=off
  PS-Simulink Converter9 : nesl_utility/PS-Simulink Converter  PhysicalDomain=network_engine_domain  SubClassName=ps_output  LeftPortType=input  RightPortType=output  PseudoPeriodic=off  Frequencies=[]  VectorFormat=inherit  Unit=inherit  AffineConversion=off
  Radians to Degrees1 : simulink_extras/Transformations/Radians to Degrees
  Radians to Degrees2 : simulink_extras/Transformations/Radians to Degrees
  Radians to Degrees4 : simulink_extras/Transformations/Radians to Degrees
  Conn1 : PMIOPort  Side=Right
  Conn2 : PMIOPort  Port=2  Side=Left
  L1-S1 FE Simscape Rotation : Outport
  L1-S1 FE Simscape Moment : Outport  Port=2
  L1-S1 LB Simscape Rotation : Outport  Port=3
  L1-S1 LB Simscape Moment : Outport  Port=4
  L1-S1 AR Simscape Rotation : Outport  Port=5
  L1-S1 AR Simscape Moment : Outport  Port=6
  wires:
  Gain5/1 -> L1-S1 AR Simscape Rotation/1  "L1-S1 AR Simscape Rotation"
  Radians to Degrees4/1 -> Add/1
  Gain3/1 -> L1-S1 LB Simscape Rotation/1  "L1-S1 LB Simscape Rotation"
  Add2/1 -> Gain5/1
  Gain8/1 -> L1-S1 AR Simscape Moment/1  "L1-S1 AR Simscape Moment"
  Gain4/1 -> L1-S1 LB Simscape Moment/1  "L1-S1 LB Simscape Moment"
  Constant2/1 -> Add/2
  PS-Simulink Converter5/1 -> Radians to Degrees2/1
  Add/1 -> Gain6/1
  Constant3/1 -> Add1/2
  Radians to Degrees1/1 -> Add1/1
  Gain7/1 -> L1-S1 FE Simscape Moment/1  "L1-S1 FE Simscape Moment"
  Radians to Degrees2/1 -> Add2/1
  Gain6/1 -> L1-S1 FE Simscape Rotation/1  "L1-S1 FE Simscape Rotation"
  Constant4/1 -> Add2/2
  In3/1 -> Gain8/1
  PS-Simulink Converter1/1 -> Radians to Degrees1/1
  In1/1 -> Gain7/1
  In2/1 -> Gain4/1
  PS-Simulink Converter9/1 -> Radians to Degrees4/1
  Add1/1 -> Gain3/1
  connections:
  PS-Simulink Converter5/LConn1 -- L1-S1 Bushing Joint/RConn4
  PS-Simulink Converter1/LConn1 -- L1-S1 Bushing Joint/RConn3
  L1-S1 Bushing Joint/LConn1 -- Conn2/RConn1
  L1-S1 Bushing Joint/RConn2 -- PS-Simulink Converter9/LConn1
  Conn1/RConn1 -- L1-S1 Bushing Joint/RConn1
